simulink library "srfPllLib"  (R2026a)
settings: Solver=VariableStepAuto
settings Model: Creator=aqiba  LastModifiedBy=aqiba

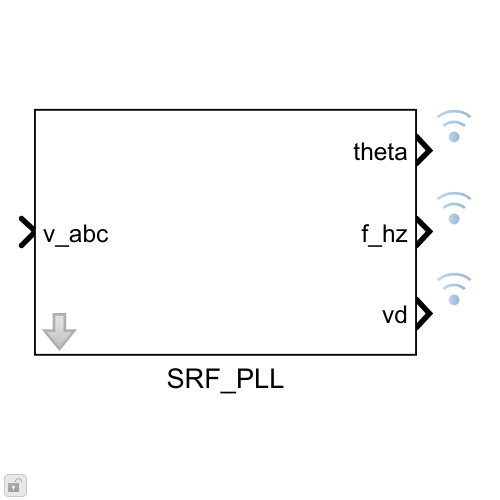
[thumbnail: Simulink's stored preview of the top-level diagram]
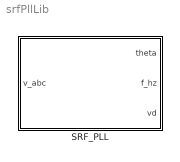
== system srfPllLib ==
  SRF_PLL : Subsystem  mask(SRF-PLL){Ts=1e-4, f0=50, fbw=25, zeta=0.707}
      mask prompts: Ts "Sample time (s)"; f0 "Nominal grid frequency (Hz)"; fbw "Loop natural frequency (Hz)"; zeta "Loop damping"
      mask help:
      | Synchronous-reference-frame PLL. In: v_abc [3x1]. Out: theta (rad, atan2 convention as GridAngle_ideal), f_hz, vd (V, grid voltage amplitude).
      | Drop-in replacement for GridAngle_ideal (use output 1).

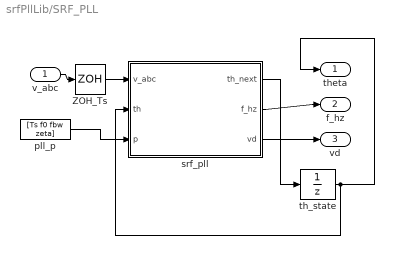
== system srfPllLib/SRF_PLL ==
  v_abc : Inport
  ZOH_Ts : ZeroOrderHold  SampleTime=Ts
  pll_p : Constant  Value=[Ts f0 fbw zeta]
  srf_pll : MATLAB Function  TreatAsAtomicUnit=on
  th_state : UnitDelay  SampleTime=Ts
  theta : Outport
  f_hz : Outport  Port=2
  vd : Outport  Port=3
  wires:
  srf_pll/3(vd) -> vd/1
  srf_pll/2(f_hz) -> f_hz/1
  pll_p/1 -> srf_pll/3(p)
  v_abc/1 -> ZOH_Ts/1
  ZOH_Ts/1 -> srf_pll/1(v_abc)
  srf_pll/1(th_next) -> th_state/1
  th_state/1 -> theta/1, srf_pll/2(th)

== matlab function srfPllLib/SRF_PLL/srf_pll ==
  data: v_abc input; th input; th_next output; p input; f_hz output; vd output
function [th_next, f_hz, vd] = srf_pll(v_abc, th, p)
% Synchronous-reference-frame PLL.  p = [Ts f0 fbw zeta]
%   Clarke -> Park at the estimated angle -> normalised vq -> 300 Hz notch
%   -> PI -> frequency (clamped f0 +/- 10 Hz) -> integrate to angle.
% theta follows GridAngle_ideal: atan2(v_beta, v_alpha), wrapped to (-pi, pi].
% th is the current estimate, held in the Unit Delay th_state outside this
% function; theta is taken from that delay, so v_abc has no direct path to theta.
persistent integ x1 x2 y1 y2
if isempty(integ), integ = 0; x1 = 0; x2 = 0; y1 = 0; y2 = 0; end
Ts = p(1); w0 = 2*pi*p(2); wn = 2*pi*p(3); zeta = p(4);
Kp = 2*zeta*wn; Ki = wn^2; wlim = 2*pi*10;
v_al = (2/3)*(v_abc(1) - 0.5*v_abc(2) - 0.5*v_abc(3));
v_be = (2/3)*(sqrt(3)/2)*(v_abc(2) - v_abc(3));
vd =  v_al*cos(th) + v_be*sin(th);
vq = -v_al*sin(th) + v_be*cos(th);
e = vq/max(sqrt(v_al^2 + v_be^2), 1e-3);      % ~ sin(angle error), voltage-independent
% notch at 6*f0: 5th and 7th grid harmonics both land at 300 Hz in the dq frame
wN = 2*pi*6*p(2); Q = 1; K = wN/tan(wN*Ts/2);
a0 = K^2 + (wN/Q)*K + wN^2;
b0 = (K^2 + wN^2)/a0; b1 = 2*(wN^2 - K^2)/a0; a1 = b1; a2 = (K^2 - (wN/Q)*K + wN^2)/a0;
ef = b0*e + b1*x1 + b0*x2 - a1*y1 - a2*y2;
x2 = x1; x1 = e; y2 = y1; y1 = ef;
% PI with frequency clamp and conditional integration (anti-windup)
integ_new = integ + Ki*Ts*ef;
w_un = w0 + Kp*ef + integ_new;
w = min(max(w_un, w0 - wlim), w0 + wlim);
if w == w_un, integ = integ_new; end
f_hz = w/(2*pi);
th_next = mod(th + w*Ts + pi, 2*pi) - pi;
